simulink model "THEGOODONEsim"  (R2022a)
settings: Solver=VariableStepAuto  StartTime=0.0  StopTime=6000  RelTol=1e-3  EnableMultiTasking=on
values from neighbouring files (symbols this model uses):
  CD_datum = Datum(:,6)    [THEGOODONE.m]
  CL_datum = Datum(:,3)    [THEGOODONE.m]
  Cm_datum = Datum(:,9)    [THEGOODONE.m]
  dCD_elev = [dCD_n5, dCD_n3, dCD_0, dCD_p3, dCD_p5]    [THEGOODONE.m]
  dCL_elev = [dCL_n5, dCL_n3, dCL_0, dCL_p3, dCL_p5]    [THEGOODONE.m]
  dCm_elev = [dCm_n5, dCm_n3, dCm_0, dCm_p3, dCm_p5]    [THEGOODONE.m]
libraries: aerolibasang x2, shared6dof x1, aerolibadyn x1, aerolibconvert2 x1
settings Model: Creator=davidrwilliams  LastModifiedBy=eyob
settings SolverCC: AlgebraicLoopSolver=TrustRegion
settings DataIOCC: LimitDataPoints=on  ReturnWorkspaceOutputs=off
settings OptimizationCC: LifeSpan=inf
settings DebuggingCC: UnconnectedInputMsg=warning  UnconnectedOutputMsg=warning  UnconnectedLineMsg=warning  AllowSymbolicDim=off  SFUnexpectedBacktrackingDiag=warning  SFNoUnconditionalDefaultTransitionDiag=warning  SFExecutionAtInitializationDiag=none  SFMachineParentedDataDiag=warning  ArithmeticOperatorsInVariantConditions=warning
settings ModelReferenceCC: PropagateSignalLabelsOutOfModel=off
settings SFSimCC: SimUseLocalCustomCode=off  CustomCodeUndefinedFunction=UseInterfaceOnly
settings RTWCC: RTWUseLocalCustomCode=off
settings CodeAppCC: StateflowObjectComments=on
settings GRTTargetCC: TargetLangStandard=C89/C90 (ANSI)
settings ConfigComp: CovMetricSettings=dw  CovSaveCumulativeToWorkspaceVar=on  CovSaveSingleToWorkspaceVar=on  CovExternalEMLEnable=off

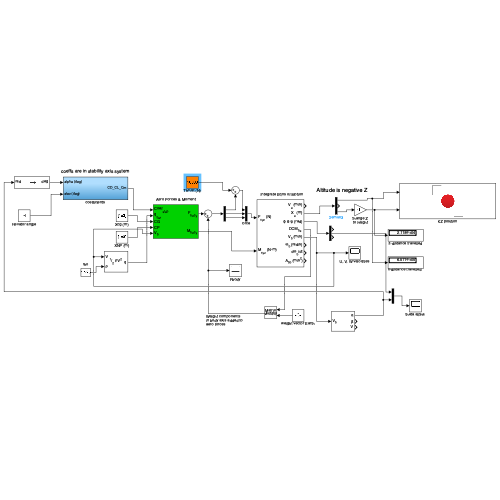
[thumbnail: Simulink's stored preview of the top-level diagram]
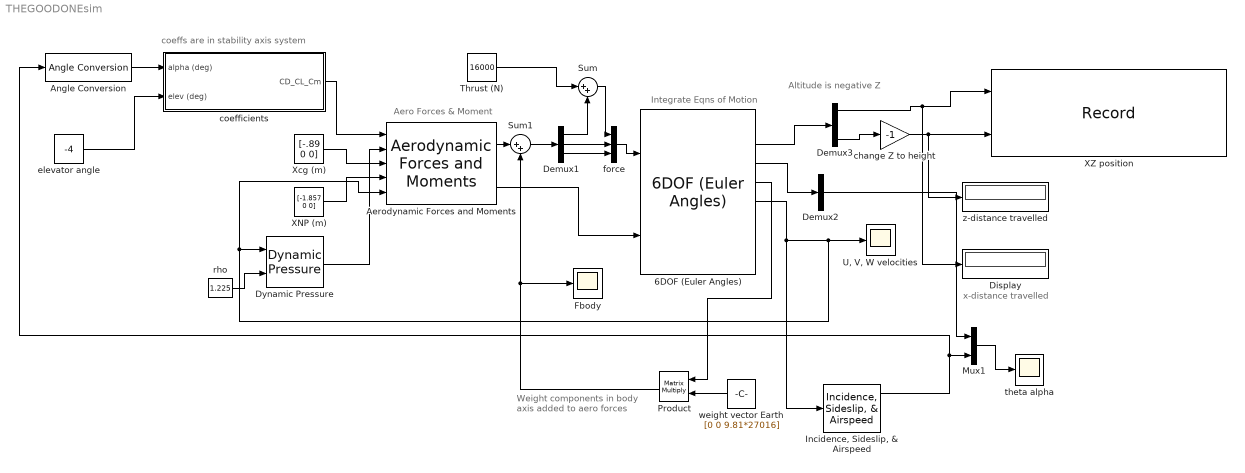
== system THEGOODONEsim ==
  note: Weight components
      | in body axis added to
      | aero forces
  note: x-distance travelled
  note: Integrate Eqns of Motion
  note: Aero Forces & Moment
  note: Altitude is negative Z
  note: coeffs are in stability axis system
  6DOF (Euler Angles) : shared6dof/6DOF (Euler Angles)  units=Metric (MKS)  mtype=Fixed  rep=Euler Angles  xme_0=[0 0 -5000]  Vm_0=[90 0 0]  eul_0=[0 0 0]  pm_0=[0 0 0]  mass_0=27016  mass_e=0.5  mass_f=2.0  inertia=[229042, 0, 1531691; 0, 1445406,0; 0, 0, 264144]  inertia_e=eye(3)  inertia_f=2*eye(3)  k_quat=1.0  vre_flag=on  abi_flag=off  aMode=0  xme_statename=''  Vm_statename=''  eul_statename=''  quat_statename=''  pm_statename=''  mass_statename=''
      settings: SourceProductBaseCode=AE,PW,DR,MT,VE
  "Aerodynamic Forces and Moments " : aerolibadyn/Aerodynamic Forces and Moments   inputAxes=Stability  outputForceAxes=Body  outputMomentAxes=Body  S=75.6  b=30.54  cbar=2.59
  Angle Conversion : aerolibconvert2/Angle Conversion  IU=rad  OU=deg
  Demux1 : Demux  Outputs=3
  Demux2 : Demux  Outputs=3
  Demux3 : Demux  Outputs=3
  Display : Display
  Dynamic Pressure : aerolibasang/Dynamic Pressure
  Fbody : Scope
  "Incidence, Sideslip, & Airspeed" : aerolibasang/Incidence, Sideslip, & Airspeed
  Mux1 : Mux  Inputs=2
  Product : Product  Multiplication=Matrix(*)
  Sum : Sum  Inputs=|++
  Sum1 : Sum  Inputs=|++
  Thrust (N) : Constant  Value=16000
  "U, V, W velocities" : Scope
  XNP (m) : Constant  Value=[-1.857 0 0]
  "XZ position " : Record  FileSettingsInternal="{\"entries\":[{\"content\":{\"excelSettings\":{\"content\":{},\"type\":\"Streamout.ExcelSettings\"}},\"type\":\"Streamout.FileSettingStorage\",\"uuid\":\"b9f9cbc5-7733-443a-ba1b-f2324a4208e9\"}],\"packageUris\":[\"http://schema.mathworks.com/mf0/streamout_blocks/R2020a\"],\"version\":\"1.0\"}"  Layout=[1 1]  SignalsInternal="{\"entries\":[{\"content\":{\"signals\":[{\"content\":{\"blockPath\":[\"THEGOODONEsim/XZ position \"],\"channel\":[],\"dimensions\":[1],\"domain\":\"THEGOODONEsim/XZ position \",\"lineColor\":\"#a2142f\",\"plots\":[1],\"port\":1,\"sid\":[\"\"],\"signalID\":1283,\"signalName\":\"Demux3:1\"},\"type\":\"RecordBlkView.Signal\",\"uuid\":\"c77b9682-5010-4b01-8eab-2b3616e88310\"},{\"content\":{\"blockPath\":[\"THEGOODONEsim/XZ position \"],\"channel\":[],\"dimensions\":[1],\"domain\":\"THEGOODONEsim/XZ position \",\"lineColor\":\"#139fff\",\"plots\":[1],\"port\":2,\"sid\":[\"\"],\"signalID\":1287,\"signalName\":\"change Z \\nto height\"},\"type\":\"RecordBlkView.Signal\",\"uuid\":\"72df68f2-9e0b-4025-83a8-26a0d0edeb42\"}]},\"type\":\"RecordBlkView.InputSignals\",\"uuid\":\"ca1d89e6-57b8-4f34-87f6-4641da943a80\"}],\"packageUris\":[\"http://schema.mathworks.com/mf0/streamout_blocks/R2020a\"],\"version\":\"1.0\"}"  VisualizationBindings="{\"xyplotplugin\":{\"info\":[{\"series\":[{\"bindingParametersList\":[{\"parameter\":\"X-Axis\",\"signalID\":1283,\"signalName\":\"Demux3:1\"},{\"parameter\":\"Y-Axis\",\"signalID\":1287,\"signalName\":\"change Z \\nto height\"}],\"seriesID\":55724}],\"subplotID\":1}]}}"  CompatibilityTag=XY  st=-1
  Xcg (m) : Constant  Value=[-.89 0 0]
  change Z to height : Gain  Gain=-1
  coefficients : Subsystem
  elevator angle : Constant  Value=-4
  force : Mux  Inputs=3
  rho : Constant  Value=1.225
  theta alpha : Scope
  weight vector Earth : Constant  Value=[0 0 9.81*27016]
  z-distance travelled : Display
  wires:
  rho/1 -> Dynamic Pressure/2
  Dynamic Pressure/1 -> "Aerodynamic Forces and Moments "/2
  Demux1/3 -> force/3
  Xcg (m)/1 -> "Aerodynamic Forces and Moments "/3
  XNP (m)/1 -> "Aerodynamic Forces and Moments "/4
  coefficients/1(CD_CL_Cm) -> "Aerodynamic Forces and Moments "/1
  Demux3/1 -> "XZ position "/1, Display/1
  Demux1/1 -> Sum/2
  Thrust (N)/1 -> Sum/1
  Angle Conversion/1 -> coefficients/1(alpha (deg))
  change Z to height/1 -> z-distance travelled/1, "XZ position "/2
  elevator angle/1 -> coefficients/2(elev (deg))
  "Incidence, Sideslip, & Airspeed"/1 -> Mux1/2, Angle Conversion/1
  Mux1/1 -> theta alpha/1
  force/1 -> 6DOF (Euler Angles)/1
  Sum/1 -> force/1
  Demux1/2 -> force/2
  "Aerodynamic Forces and Moments "/2 -> 6DOF (Euler Angles)/2
  Demux3/3 -> change Z to height/1
  6DOF (Euler Angles)/2 -> Demux3/1
  6DOF (Euler Angles)/5 -> Dynamic Pressure/1, "Aerodynamic Forces and Moments "/5, "U, V, W velocities"/1, "Incidence, Sideslip, & Airspeed"/1
  6DOF (Euler Angles)/3 -> Demux2/1
  Demux2/2 -> Mux1/1
  weight vector Earth/1 -> Product/2
  6DOF (Euler Angles)/4 -> Product/1
  "Aerodynamic Forces and Moments "/1 -> Sum1/1
  Sum1/1 -> Demux1/1
  Product/1 -> Fbody/1, Sum1/2

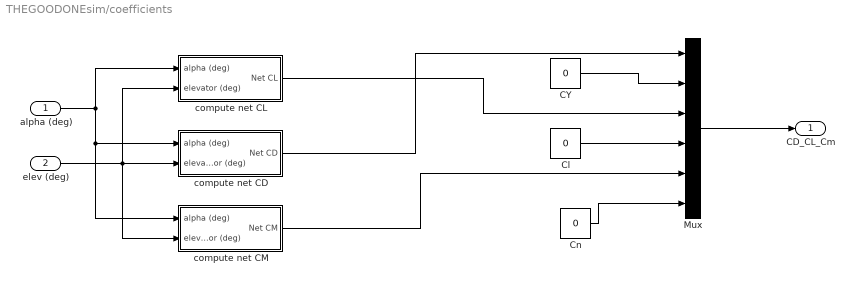
== system THEGOODONEsim/coefficients ==
  alpha (deg) : Inport
  elev (deg) : Inport  Port=2
  CY : Constant  Value=0
  Cl : Constant  Value=0
  Cn : Constant  Value=0
  Mux : Mux  Inputs=6
  compute net CD : Subsystem
  compute net CL : Subsystem
  compute net CM : Subsystem
  CD_CL_Cm : Outport
  wires:
  CY/1 -> Mux/2
  Cl/1 -> Mux/4
  Cn/1 -> Mux/6
  Mux/1 -> CD_CL_Cm/1
  elev (deg)/1 -> compute net CD/2(elevator (deg)), compute net CM/2(elevator (deg)), compute net CL/2(elevator (deg))
  alpha (deg)/1 -> compute net CD/1(alpha (deg)), compute net CM/1(alpha (deg)), compute net CL/1(alpha (deg))
  compute net CD/1(Net CD) -> Mux/1
  compute net CL/1(Net CL) -> Mux/3
  compute net CM/1(Net CM) -> Mux/5

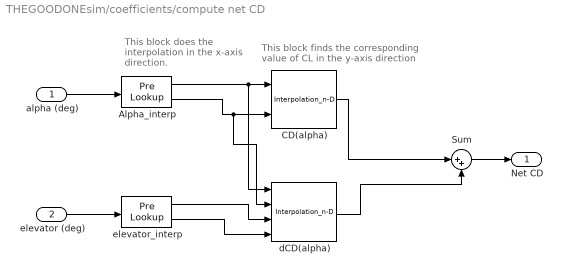
== system THEGOODONEsim/coefficients/compute net CD ==
  note: This block finds the corresponding
      | value of CL in the y-axis direction
  note: This block does the interpolation in the
      | x-axis direction.
  alpha (deg) : Inport
  elevator (deg) : Inport  Port=2
  Alpha_interp : PreLookup  BreakpointsData=alpha  BeginIndexSearchUsingPreviousIndexResult=on  ExtrapMethod=Linear
  CD(alpha) : Interpolation_n-D  NumberOfTableDimensions=1  Table=CD_datum  RemoveProtectionIndex=on
      settings: InputPortMap=u0,u1
  Sum : Sum  Inputs=|++
  dCD(alpha) : Interpolation_n-D  Table=dCD_elev  RemoveProtectionIndex=on
  elevator_interp : PreLookup  BreakpointsData=delev  BeginIndexSearchUsingPreviousIndexResult=on  ExtrapMethod=Linear
  Net CD : Outport
  wires:
  Alpha_interp/1 -> dCD(alpha)/1, CD(alpha)/1
  Alpha_interp/2 -> dCD(alpha)/2, CD(alpha)/2
  CD(alpha)/1 -> Sum/1
  alpha (deg)/1 -> Alpha_interp/1
  elevator (deg)/1 -> elevator_interp/1
  elevator_interp/2 -> dCD(alpha)/4
  elevator_interp/1 -> dCD(alpha)/3
  dCD(alpha)/1 -> Sum/2
  Sum/1 -> Net CD/1

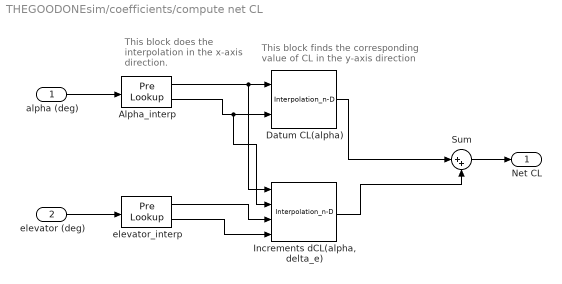
== system THEGOODONEsim/coefficients/compute net CL ==
  note: This block finds the corresponding
      | value of CL in the y-axis direction
  note: This block does the interpolation in the
      | x-axis direction.
  alpha (deg) : Inport
  elevator (deg) : Inport  Port=2
  Alpha_interp : PreLookup  BreakpointsData=alpha  BeginIndexSearchUsingPreviousIndexResult=on  ExtrapMethod=Linear
  Datum CL(alpha) : Interpolation_n-D  NumberOfTableDimensions=1  Table=CL_datum  RemoveProtectionIndex=on
      settings: InputPortMap=u0,u1
  "Increments dCL(alpha, delta_e)" : Interpolation_n-D  Table=dCL_elev  RemoveProtectionIndex=on
  Sum : Sum  Inputs=|++
  elevator_interp : PreLookup  BreakpointsData=delev  BeginIndexSearchUsingPreviousIndexResult=on  ExtrapMethod=Linear
  Net CL : Outport
  wires:
  Alpha_interp/1 -> "Increments dCL(alpha, delta_e)"/1, Datum CL(alpha)/1
  Alpha_interp/2 -> "Increments dCL(alpha, delta_e)"/2, Datum CL(alpha)/2
  Datum CL(alpha)/1 -> Sum/1
  alpha (deg)/1 -> Alpha_interp/1
  elevator (deg)/1 -> elevator_interp/1
  elevator_interp/2 -> "Increments dCL(alpha, delta_e)"/4
  elevator_interp/1 -> "Increments dCL(alpha, delta_e)"/3
  "Increments dCL(alpha, delta_e)"/1 -> Sum/2
  Sum/1 -> Net CL/1

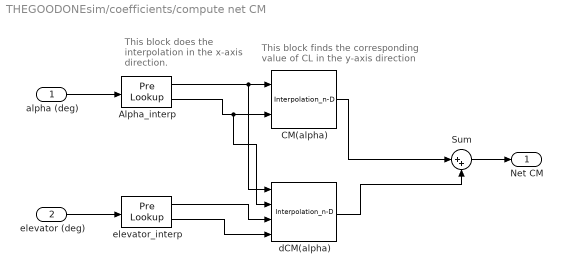
== system THEGOODONEsim/coefficients/compute net CM ==
  note: This block finds the corresponding
      | value of CL in the y-axis direction
  note: This block does the interpolation in the
      | x-axis direction.
  alpha (deg) : Inport
  elevator (deg) : Inport  Port=2
  Alpha_interp : PreLookup  BreakpointsData=alpha  BeginIndexSearchUsingPreviousIndexResult=on  ExtrapMethod=Linear
  CM(alpha) : Interpolation_n-D  NumberOfTableDimensions=1  Table=Cm_datum  RemoveProtectionIndex=on
      settings: InputPortMap=u0,u1
  Sum : Sum  Inputs=|++
  dCM(alpha) : Interpolation_n-D  Table=dCm_elev  RemoveProtectionIndex=on
  elevator_interp : PreLookup  BreakpointsData=delev  BeginIndexSearchUsingPreviousIndexResult=on  ExtrapMethod=Linear
  Net CM : Outport
  wires:
  Alpha_interp/1 -> dCM(alpha)/1, CM(alpha)/1
  Alpha_interp/2 -> dCM(alpha)/2, CM(alpha)/2
  CM(alpha)/1 -> Sum/1
  alpha (deg)/1 -> Alpha_interp/1
  elevator (deg)/1 -> elevator_interp/1
  elevator_interp/2 -> dCM(alpha)/4
  elevator_interp/1 -> dCM(alpha)/3
  dCM(alpha)/1 -> Sum/2
  Sum/1 -> Net CM/1
